simulink model "wam_sim"  (Simulink 9.2)
settings: Solver=ode45  StartTime=0.0  StopTime=10  RelTol=1e-3  EnableMultiTasking=on
values from neighbouring files (symbols this model uses):
  Z0 = [0;0;0;0;0;0]    [parameter_cal.m]
undefined symbols (not defined in the file or in its folder): robust_passivity, stateder
settings Model: Creator=rhanz  LastModifiedBy=arsh  ExtModeAutoUpdateStatusClock=off
settings OptimizationCC: InitFltsAndDblsToZero=on
settings DebuggingCC: SaveWithParameterizedLinksMsg=none  SignalResolutionControl=TryResolveAllWithWarning  SolverPrmCheckMsg=warning  MultiTaskDSMMsg=warning  MultiTaskCondExecSysMsg=none  StateNameClashWarn=none
settings SFSimCC: SimUseLocalCustomCode=on
settings RTWCC: RTWUseLocalCustomCode=on
settings GRTTargetCC: TargetFcnLib=ansi_tfl_tmw.mat  GeneratePreprocessorConditionals=Use local settings
settings ConfigComp: CovExternalEMLEnable=on

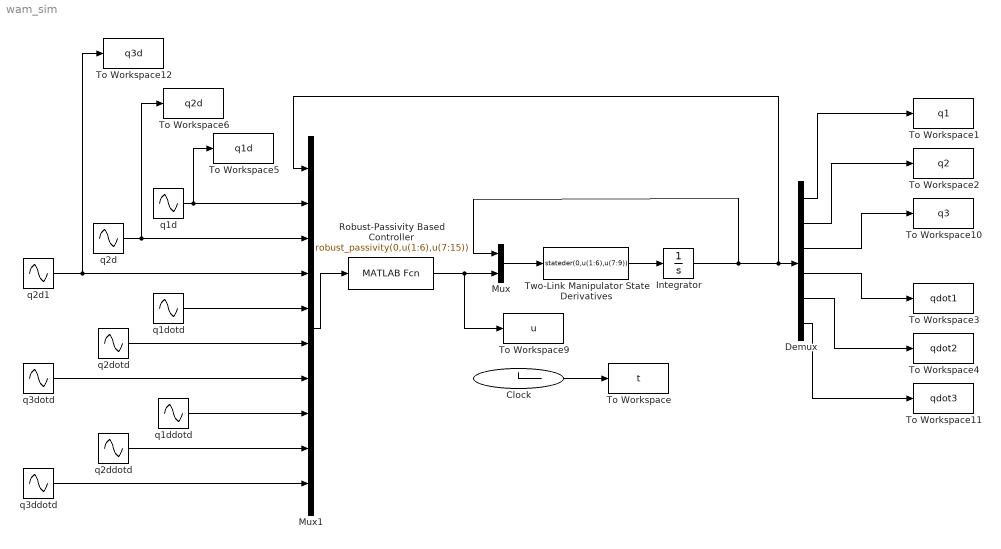
== system wam_sim ==
  Clock : Clock
  Demux : Demux  Outputs=6
  Integrator : Integrator  InitialCondition=Z0
  Mux : Mux  Inputs=2
  Mux1 : Mux  Inputs=10
  Robust-Passivity Based Controller : MATLABFcn  MATLABFcn=robust_passivity(0,u(1:6),u(7:15))  OutputDimensions=3
  To Workspace : ToWorkspace  VariableName=t  SampleTime=-1
  To Workspace1 : ToWorkspace  VariableName=q1  SampleTime=-1
  To Workspace10 : ToWorkspace  VariableName=q3  SampleTime=-1
  To Workspace11 : ToWorkspace  VariableName=qdot3  SampleTime=-1
  To Workspace12 : ToWorkspace  VariableName=q3d  SampleTime=-1
  To Workspace2 : ToWorkspace  VariableName=q2  SampleTime=-1
  To Workspace3 : ToWorkspace  VariableName=qdot1  SampleTime=-1
  To Workspace4 : ToWorkspace  VariableName=qdot2  SampleTime=-1
  To Workspace5 : ToWorkspace  VariableName=q1d  SampleTime=-1
  To Workspace6 : ToWorkspace  VariableName=q2d  SampleTime=-1
  To Workspace9 : ToWorkspace  VariableName=u  SampleTime=-1
  Two-Link Manipulator State Derivatives : MATLABFcn  MATLABFcn=stateder(0,u(1:6),u(7:9))  OutputDimensions=6
  q1d : Sin  SampleTime=0
  q1ddotd : Sin  Phase=pi  SampleTime=0
  q1dotd : Sin  Phase=pi/2  SampleTime=0
  q2d : Sin  Bias=-0.5  SampleTime=0
  q2d1 : Sin  Amplitude=0.75  SampleTime=0
  q2ddotd : Sin  Phase=pi  SampleTime=0
  q2dotd : Sin  Phase=pi/2  SampleTime=0
  q3ddotd : Sin  Amplitude=0.75  Phase=pi  SampleTime=0
  q3dotd : Sin  Amplitude=0.75  Phase=pi/2  SampleTime=0
  wires:
  Two-Link Manipulator State Derivatives/1 -> Integrator/1
  Integrator/1 -> Mux/1, Mux1/1, Demux/1
  Mux/1 -> Two-Link Manipulator State Derivatives/1
  Clock/1 -> To Workspace/1
  Demux/1 -> To Workspace1/1
  Demux/2 -> To Workspace2/1
  Demux/5 -> To Workspace4/1
  Robust-Passivity Based Controller/1 -> To Workspace9/1, Mux/2
  Mux1/1 -> Robust-Passivity Based Controller/1
  q1d/1 -> Mux1/2, To Workspace5/1
  q2d/1 -> To Workspace6/1, Mux1/3
  q1dotd/1 -> Mux1/5
  q2dotd/1 -> Mux1/6
  q1ddotd/1 -> Mux1/8
  q2ddotd/1 -> Mux1/9
  Demux/4 -> To Workspace3/1
  Demux/3 -> To Workspace10/1
  Demux/6 -> To Workspace11/1
  q2d1/1 -> To Workspace12/1, Mux1/4
  q3dotd/1 -> Mux1/7
  q3ddotd/1 -> Mux1/10
